simulink model "CowleyLabExperiment1"  (R2022b)
settings: Solver=FixedStepAuto  StartTime=0.0  StopTime=100  FixedStep=0.001  RelTol=1e-3
values from neighbouring files (symbols this model uses):
  c = wn^2    [poleIdentification.m]    (also in tfCharacterisitcs.m = 4)
  m = 0.5    [Cowley_436HW2.m]
settings Model: Creator=rmdsouza  LastModifiedBy=mattcowley
settings SolverCC: AlgebraicLoopSolver=TrustRegion
settings DataIOCC: LimitDataPoints=on  SaveFormat=Array  ReturnWorkspaceOutputs=off
settings OptimizationCC: LifeSpan=inf
settings DebuggingCC: UnconnectedInputMsg=warning  UnconnectedOutputMsg=warning  UnconnectedLineMsg=warning  SFUnexpectedBacktrackingDiag=warning  SFNoUnconditionalDefaultTransitionDiag=warning  SFExecutionAtInitializationDiag=none  SFMachineParentedDataDiag=warning  ArithmeticOperatorsInVariantConditions=warning
settings HardwareCC: ProdBitPerPointer=32  ProdBitPerSizeT=32  ProdBitPerPtrDiffT=32  ProdLargestAtomicFloat=None  ProdIntDivRoundTo=Undefined  ProdEndianess=Unspecified  ProdWordSize=32  ProdHWDeviceType=32-bit Generic
settings ModelReferenceCC: EnableRefExpFcnMdlSchedulingChecks=on  PropagateSignalLabelsOutOfModel=off
settings SFSimCC: SimUseLocalCustomCode=off  CustomCodeUndefinedFunction=UseInterfaceOnly
settings RTWCC: RTWUseLocalCustomCode=off
settings CodeAppCC: StateflowObjectComments=on
settings GRTTargetCC: TargetLangStandard=C89/C90 (ANSI)
settings ConfigComp: CovMetricSettings=dw  CovSaveCumulativeToWorkspaceVar=on  CovSaveSingleToWorkspaceVar=on  CovExternalEMLEnable=off

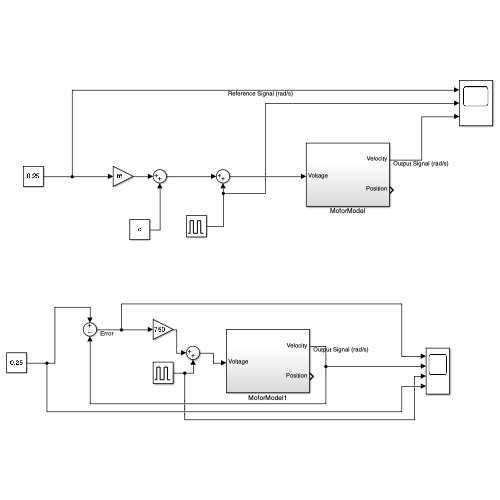
[thumbnail: Simulink's stored preview of the top-level diagram]
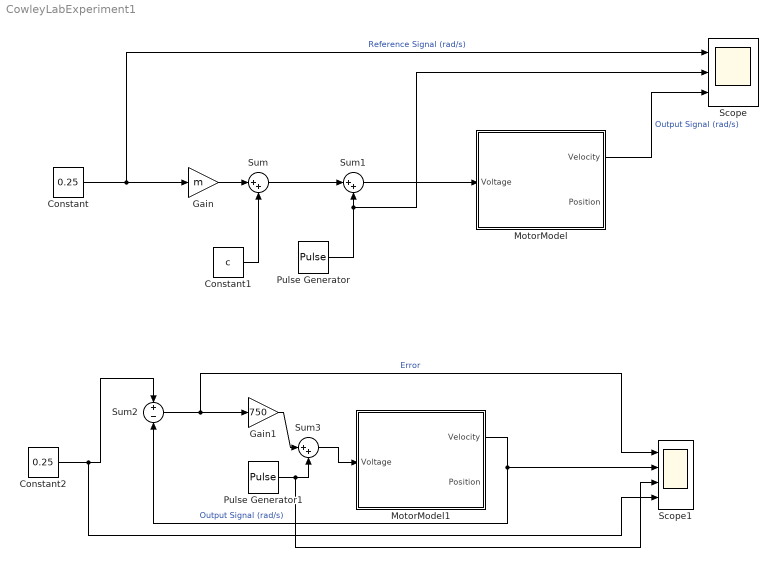
== system CowleyLabExperiment1 ==
  Constant : Constant  Value=0.25
  Constant1 : Constant  Value=c
  Constant2 : Constant  Value=0.25
  Gain : Gain  Gain=m
  Gain1 : Gain  Gain=750
  MotorModel : Subsystem
  MotorModel1 : Subsystem
  Pulse Generator : DiscretePulseGenerator  PulseType=Time based  Amplitude=0.25  Period=10  PulseWidth=50
  Pulse Generator1 : DiscretePulseGenerator  PulseType=Time based  Amplitude=0.25  Period=10  PulseWidth=50
  Scope : Scope  NumInputPorts=3
  Scope1 : Scope  NumInputPorts=4
  Sum : Sum  Inputs=|++
  Sum1 : Sum  Inputs=|++
  Sum2 : Sum  Inputs=+-
  Sum3 : Sum  Inputs=|++
  wires:
  Constant/1 -> Scope/1, Gain/1  "Reference Signal (rad/s)"
  Constant1/1 -> Sum/2
  Gain/1 -> Sum/1
  MotorModel/1(Velocity) -> Scope/3  "Output Signal (rad/s)"
  Pulse Generator/1 -> Scope/2, Sum1/2
  Sum/1 -> Sum1/1
  Sum1/1 -> MotorModel/1(Voltage)
  MotorModel1/1(Velocity) -> Sum2/2, Scope1/2  "Output Signal (rad/s)"
  Constant2/1 -> Scope1/4, Sum2/1
  Sum2/1 -> Scope1/1, Gain1/1  "Error"
  Pulse Generator1/1 -> Scope1/3, Sum3/2
  Gain1/1 -> Sum3/1
  Sum3/1 -> MotorModel1/1(Voltage)

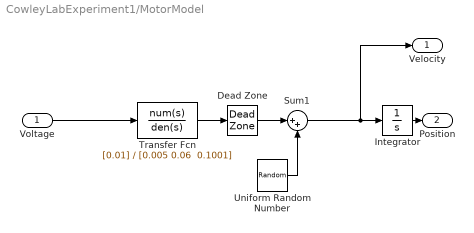
== system CowleyLabExperiment1/MotorModel ==
  Voltage : Inport
  Dead Zone : DeadZone  LowerValue=-0.1  UpperValue=0.1
  Integrator : Integrator
  Sum1 : Sum  Inputs=|++
  Transfer Fcn : TransferFcn  Numerator=[0.01]  Denominator="[0.005 0.06  0.1001]"
  Uniform Random Number : UniformRandomNumber  Minimum=-0.005  Maximum=0.005  SampleTime=0.01
  Velocity : Outport
  Position : Outport  Port=2
  wires:
  Voltage/1 -> Transfer Fcn/1
  Integrator/1 -> Position/1
  Transfer Fcn/1 -> Dead Zone/1
  Dead Zone/1 -> Sum1/1
  Uniform Random Number/1 -> Sum1/2
  Sum1/1 -> Integrator/1, Velocity/1

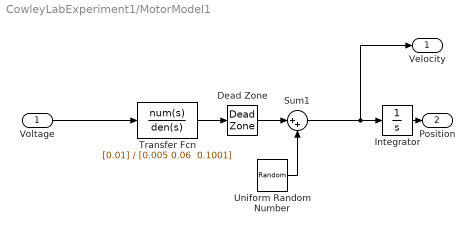
== system CowleyLabExperiment1/MotorModel1 ==
  Voltage : Inport
  Dead Zone : DeadZone  LowerValue=-0.1  UpperValue=0.1
  Integrator : Integrator
  Sum1 : Sum  Inputs=|++
  Transfer Fcn : TransferFcn  Numerator=[0.01]  Denominator="[0.005 0.06  0.1001]"
  Uniform Random Number : UniformRandomNumber  Minimum=-0.005  Maximum=0.005  SampleTime=0.01
  Velocity : Outport
  Position : Outport  Port=2
  wires:
  Voltage/1 -> Transfer Fcn/1
  Integrator/1 -> Position/1
  Transfer Fcn/1 -> Dead Zone/1
  Dead Zone/1 -> Sum1/1
  Uniform Random Number/1 -> Sum1/2
  Sum1/1 -> Integrator/1, Velocity/1
